simulink model "Have_Loop_Current"  (Simulink 7.5)
settings: Solver=ode45  StartTime=0.0  StopTime=10  RelTol=1e-3
libraries: powerlib x28, simulink x2, powerlib_extras x2
settings Model: Creator=lm  LastModifiedBy=lm

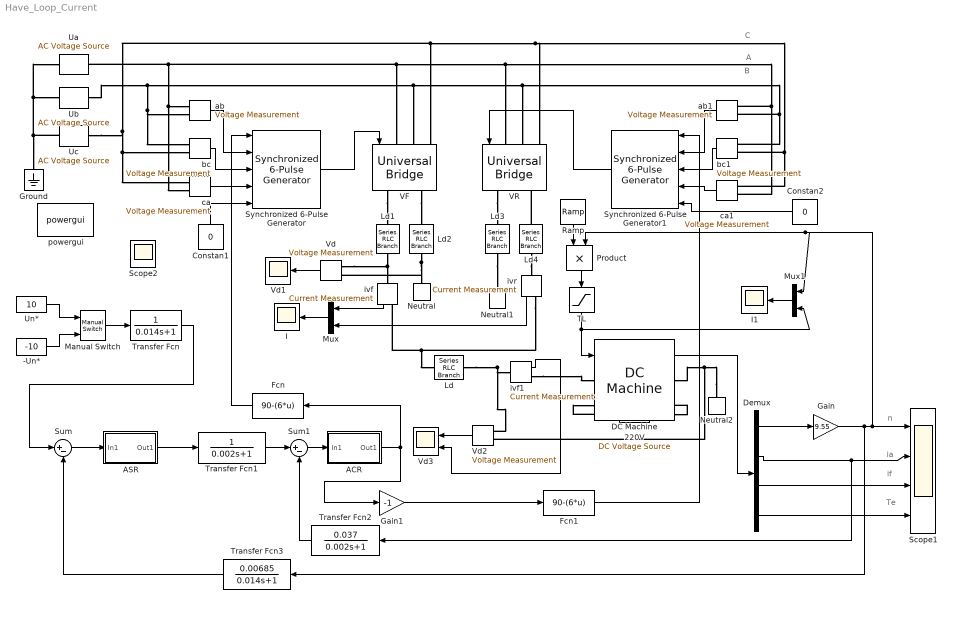
== system Have_Loop_Current ==
  note: A
  note: B
  note: C
  note: n
  note: ia
  note: if
  note: Te
  -Un* : Constant  Value=-10  OutDataType=fixdt(1, 16)  OutScaling=2^0
  220V : powerlib/Electrical Sources/DC Voltage Source  DialogController=POWERSYS.PowerSysDialog  SystemSampleTime=-1  Amplitude=220  Measurements=None
  ACR : Subsystem
  ASR : Subsystem
  Constan1 : Constant  Value=0  OutDataType=fixdt(1, 16)  OutScaling=2^0
  Constan2 : Constant  Value=0  OutDataType=fixdt(1, 16)  OutScaling=2^0
  DC Machine : powerlib/Machines/DC Machine  DialogController=POWERSYS.PowerSysDialog  SystemSampleTime=-1  PresetModel=No  MechanicalLoad=Torque TL  FieldType=Wound  ShowDetailedParameters=on  RLa="[ 0.21  0.000543]"  RLf="[ 14.7  0]"  Laf=0.084  MachineConstant=Torque constant (N.m/A)  Ke=1.8  Kt=1.8  J=2.29  Bm=0  Tf=0  w0=1  Ifinit=1  TsPowergui=0  TsBlock=-1
      settings: AttributesFormatString=\n
  Demux : Demux
  Fcn : Fcn  Expr=90-(6*u)
  Fcn1 : Fcn  Expr=90-(6*u)
  Gain : Gain  Gain=9.55  ParameterDataType=fixdt(1, 16)  ParameterScaling=2^0  OutDataType=fixdt(1, 16)  OutScaling=2^0
  Gain1 : Gain  Gain=-1  ParameterDataType=fixdt(1, 16)  ParameterScaling=2^0  OutDataType=fixdt(1, 16)  OutScaling=2^0
  Ground : powerlib/Elements/Ground  DialogController=POWERSYS.PowerSysDialog  PhysicalDomain=powersysdomain  SubClassName=unknown  LeftPortType=p1  RightPortType=p1  LConnTagsString=a
  I : Scope
  I1 : Scope
      settings: SaveName=ScopeData5
  Ld : powerlib/Elements/Series RLC Branch  DialogController=POWERSYS.PowerSysDialog  PhysicalDomain=powersysdomain  SubClassName=unknown  LeftPortType=p1  RightPortType=p1  LConnTagsString=__new0  RConnTagsString=__new0  BranchType=RL  Resistance=0.002  Inductance=0.015  SetiL0=off  InitialCurrent=0  Capacitance=1e-6  Setx0=off  InitialVoltage=0  Measurements=None
  Ld{1..4} (4 alike) : powerlib/Elements/Series RLC Branch  DialogController=POWERSYS.PowerSysDialog  PhysicalDomain=powersysdomain  SubClassName=unknown  LeftPortType=p1  RightPortType=p1  LConnTagsString=__new0  RConnTagsString=__new0  BranchType=L  Resistance=1  Inductance=2e-3  SetiL0=off  InitialCurrent=0  Capacitance=1e-6  Setx0=off  InitialVoltage=0  Measurements=None
  Manual Switch : simulink/Signal Routing/Manual Switch  SystemSampleTime=-1  sw=0  action=0  varsize=off
  Mux : Mux  Inputs=2
  Mux1 : Mux  Inputs=2
  Neutral : powerlib/Elements/Neutral  DialogController=POWERSYS.PowerSysDialog  PhysicalDomain=powersysdomain  SubClassName=unknown  LeftPortType=p1  RightPortType=p1  LConnTagsString=a  NodeNumber=10
  Neutral1 : powerlib/Elements/Neutral  DialogController=POWERSYS.PowerSysDialog  PhysicalDomain=powersysdomain  SubClassName=unknown  LeftPortType=p1  RightPortType=p1  LConnTagsString=a  NodeNumber=10
  Neutral2 : powerlib/Elements/Neutral  DialogController=POWERSYS.PowerSysDialog  PhysicalDomain=powersysdomain  SubClassName=unknown  LeftPortType=p1  RightPortType=p1  LConnTagsString=a  NodeNumber=10
  Product : Product  OutDataType=fixdt(1, 16)  OutScaling=2^0  RndMeth=Zero
  Ramp : simulink/Sources/Ramp  SystemSampleTime=-1  slope=10000  start=2.2  X0=0
  Scope1 : Scope  NumInputPorts=4
      settings: YMin=1275~-20~14.966~-25  YMax=1475~140~14.966~175
  Scope2 : Scope
      settings: YMin=-10  YMax=10  SaveName=ScopeData2
  Sum : Sum  Inputs=|+-  OutDataType=fixdt(1, 16)  OutScaling=2^0
  Sum1 : Sum  Inputs=|+-  OutDataType=fixdt(1, 16)  OutScaling=2^0
  Synchronized 6-Pulse Generator : powerlib_extras/Control  Blocks/Synchronized 6-Pulse Generator  DialogController=POWERSYS.PowerSysDialog  SystemSampleTime=-1  freq=60  pwidth=10  Double_Pulse=off
  Synchronized 6-Pulse Generator1 : powerlib_extras/Control  Blocks/Synchronized 6-Pulse Generator  DialogController=POWERSYS.PowerSysDialog  SystemSampleTime=-1  freq=60  pwidth=10  Double_Pulse=off
  TL : Saturate  UpperLimit=160  LowerLimit=-160  OutDataType=fixdt(1, 16)  OutScaling=2^0
  Transfer Fcn : TransferFcn  Denominator=[0.014 1]
  Transfer Fcn1 : TransferFcn  Denominator=[0.002 1]
  Transfer Fcn2 : TransferFcn  Numerator=[0.037]  Denominator=[0.002 1]
  Transfer Fcn3 : TransferFcn  Numerator=[0.00685]  Denominator=[0.014 1]
  Ua : powerlib/Electrical Sources/AC Voltage Source  DialogController=POWERSYS.PowerSysDialog  SystemSampleTime=-1  Amplitude=160  Phase=0  Frequency=50  SampleTime=0  Measurements=None
  Ub : powerlib/Electrical Sources/AC Voltage Source  DialogController=POWERSYS.PowerSysDialog  SystemSampleTime=-1  Amplitude=160  Phase=-120  Frequency=50  SampleTime=0  Measurements=None
  Uc : powerlib/Electrical Sources/AC Voltage Source  DialogController=POWERSYS.PowerSysDialog  SystemSampleTime=-1  Amplitude=160  Phase=-240  Frequency=50  SampleTime=0  Measurements=None
  Un* : Constant  Value=10  OutDataType=fixdt(1, 16)  OutScaling=2^0
  VF : powerlib/Power Electronics/Universal Bridge  DialogController=POWERSYS.PowerSysDialog  SystemSampleTime=-1  Arms=3  SnubberResistance=1e5  SnubberCapacitance=inf  Device=Thyristors  Ron=1e-3  Lon=0  ForwardVoltages="[  0  0  ]"  ForwardVoltage=0  GTOparameters=[ 10e-6 , 20e-6 ]  IGBTparameters=[ 1e-6 , 2e-6 ]  Measurements=None  Measurements_2=None  converterType=Rectifier
  VR : powerlib/Power Electronics/Universal Bridge  DialogController=POWERSYS.PowerSysDialog  SystemSampleTime=-1  Arms=3  SnubberResistance=1e5  SnubberCapacitance=inf  Device=Thyristors  Ron=1e-3  Lon=0  ForwardVoltages="[  0  0  ]"  ForwardVoltage=0  GTOparameters=[ 10e-6 , 20e-6 ]  IGBTparameters=[ 1e-6 , 2e-6 ]  Measurements=None  Measurements_2=None  converterType=Rectifier
  Vd : powerlib/Measurements/Voltage Measurement  DialogController=POWERSYS.PowerSysDialog  SystemSampleTime=-1  PhasorSimulation=off  OutputType=Complex  PSBequivalent=0
  Vd1 : Scope
      settings: YMin=-400  YMax=500  SaveName=ScopeData3
  Vd2 : powerlib/Measurements/Voltage Measurement  DialogController=POWERSYS.PowerSysDialog  SystemSampleTime=-1  PhasorSimulation=off  OutputType=Complex  PSBequivalent=0
  Vd3 : Scope  NumInputPorts=2
      settings: YMin=-5~-5  YMax=5~5  SaveName=ScopeData4
  ab : powerlib/Measurements/Voltage Measurement  DialogController=POWERSYS.PowerSysDialog  SystemSampleTime=-1  PhasorSimulation=off  OutputType=Complex  PSBequivalent=0
  ab1 : powerlib/Measurements/Voltage Measurement  DialogController=POWERSYS.PowerSysDialog  SystemSampleTime=-1  PhasorSimulation=off  OutputType=Complex  PSBequivalent=0
  bc : powerlib/Measurements/Voltage Measurement  DialogController=POWERSYS.PowerSysDialog  SystemSampleTime=-1  PhasorSimulation=off  OutputType=Complex  PSBequivalent=0
  bc1 : powerlib/Measurements/Voltage Measurement  DialogController=POWERSYS.PowerSysDialog  SystemSampleTime=-1  PhasorSimulation=off  OutputType=Complex  PSBequivalent=0
  ca : powerlib/Measurements/Voltage Measurement  DialogController=POWERSYS.PowerSysDialog  SystemSampleTime=-1  PhasorSimulation=off  OutputType=Complex  PSBequivalent=0
  ca1 : powerlib/Measurements/Voltage Measurement  DialogController=POWERSYS.PowerSysDialog  SystemSampleTime=-1  PhasorSimulation=off  OutputType=Complex  PSBequivalent=0
  ivf : powerlib/Measurements/Current Measurement  DialogController=POWERSYS.PowerSysDialog  SystemSampleTime=-1  PhasorSimulation=off  OutputType=Complex  PSBequivalent=0
  ivf1 : powerlib/Measurements/Current Measurement  DialogController=POWERSYS.PowerSysDialog  SystemSampleTime=-1  PhasorSimulation=off  OutputType=Complex  PSBequivalent=0
  ivr : powerlib/Measurements/Current Measurement  DialogController=POWERSYS.PowerSysDialog  SystemSampleTime=-1  PhasorSimulation=off  OutputType=Complex  PSBequivalent=0
  powergui : powerlib/powergui  Priority=1  SystemSampleTime=-1  SimulationMode=Discrete  SampleTime=50e-6  frequency=60  SPID=off  DisableSnubberDevices=off  DisableRonSwitches=off  DisableVfSwitches=off  SwTol=0  Interpol=off  frequencyindice=0  echomessages=off  HookPort=off  DisplayEquations=off  FunctionMessages=off  EnableUseOfTLC=off  x0status=blocks  RestoreLinks=warning  ResistiveCurrentMeasurement=off  Ylog=off  Xlog=on  ShowGrid=off  save=off  variable=ZData  ZoomFFT=off  StartTime=0.0  cycles=1  DisplayStyle=1  FreqAxis=off  MaxFrequency=1000  frequencyindicesteady=1  display=off  methode=off
  wires:
  ab/1 -> Synchronized 6-Pulse Generator/2
  bc/1 -> Synchronized 6-Pulse Generator/3
  ca/1 -> Synchronized 6-Pulse Generator/4
  Constan1/1 -> Synchronized 6-Pulse Generator/5
  Synchronized 6-Pulse Generator/1 -> VF/1
  Synchronized 6-Pulse Generator1/1 -> VR/1
  ab1/1 -> Synchronized 6-Pulse Generator1/2
  bc1/1 -> Synchronized 6-Pulse Generator1/3
  ca1/1 -> Synchronized 6-Pulse Generator1/4
  Constan2/1 -> Synchronized 6-Pulse Generator1/5
  Un*/1 -> Manual Switch/1
  -Un*/1 -> Manual Switch/2
  Manual Switch/1 -> Transfer Fcn/1
  DC Machine/1 -> Demux/1
  Demux/1 -> Gain/1
  Gain/1 -> Transfer Fcn3/1, Scope1/1, Product/2, Mux1/1
  Demux/2 -> Scope1/2, Transfer Fcn2/1
  Demux/3 -> Scope1/3
  Demux/4 -> Scope1/4
  Transfer Fcn/1 -> Sum/1
  ASR/1(Out1) -> Transfer Fcn1/1
  Sum/1 -> ASR/1(In1)
  Transfer Fcn1/1 -> Sum1/1
  Sum1/1 -> ACR/1(In1)
  ACR/1(Out1) -> Fcn/1, Gain1/1
  Fcn/1 -> Synchronized 6-Pulse Generator/1
  Gain1/1 -> Fcn1/1
  Fcn1/1 -> Synchronized 6-Pulse Generator1/1
  Transfer Fcn2/1 -> Sum1/2
  Transfer Fcn3/1 -> Sum/2
  ivf/1 -> Mux/1
  ivr/1 -> Mux/2
  Mux/1 -> I/1
  Vd/1 -> Vd1/1
  Vd2/1 -> Vd3/1
  ivf1/1 -> Vd3/2
  TL/1 -> DC Machine/1, Mux1/2
  Ramp/1 -> Product/1
  Product/1 -> TL/1
  Mux1/1 -> I1/1
  connections:
  Uc/LConn1 -- Ground/LConn1 -- Ub/LConn1 -- Ua/LConn1
  220V/RConn1 -- DC Machine/LConn2
  220V/LConn1 -- DC Machine/RConn2
  VF/LConn1 -- ab1/LConn1 -- ca1/LConn2 -- VR/LConn1 -- Ua/RConn1 -- ab/LConn1 -- ca/LConn2
  Ub/RConn1 -- ab/LConn2 -- bc/LConn1 -- VF/LConn2 -- ab1/LConn2 -- bc1/LConn1 -- VR/LConn2
  VF/LConn3 -- bc1/LConn2 -- ca1/LConn1 -- VR/LConn3 -- Uc/RConn1 -- bc/LConn2 -- ca/LConn1
  VF/RConn1 -- Ld1/LConn1
  VF/RConn2 -- Ld2/LConn1
  VR/RConn1 -- Ld3/LConn1
  Ld4/LConn1 -- VR/RConn2
  Vd/LConn1 -- ivf/LConn1 -- Ld1/RConn1
  ivr/RConn1 -- ivf/RConn1 -- Ld/LConn1
  Ld/RConn1 -- Vd2/LConn1 -- ivf1/LConn1
  Neutral/LConn1 -- Ld2/RConn1 -- Vd/LConn2
  Neutral2/LConn1 -- DC Machine/RConn1 -- Vd2/LConn2
  Ld4/RConn1 -- ivr/LConn1
  ivf1/RConn1 -- DC Machine/LConn1
  Ld3/RConn1 -- Neutral1/LConn1

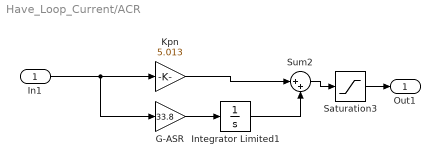
== system Have_Loop_Current/ACR ==
  In1 : Inport
  G-ASR : Gain  Gain=33.8  ParameterDataType=fixdt(1, 16)  ParameterScaling=2^0  OutDataType=fixdt(1, 16)  OutScaling=2^0
  Integrator Limited1 : Integrator  LimitOutput=on  UpperSaturationLimit=12  LowerSaturationLimit=-12
  Kpn : Gain  Gain=5.013  ParameterDataType=fixdt(1, 16)  ParameterScaling=2^0  OutDataType=fixdt(1, 16)  OutScaling=2^0
  Saturation3 : Saturate  UpperLimit=10  LowerLimit=-10  OutDataType=fixdt(1, 16)  OutScaling=2^0
  Sum2 : Sum  Inputs=|++  OutDataType=fixdt(1, 16)  OutScaling=2^0
  Out1 : Outport
  wires:
  Saturation3/1 -> Out1/1
  In1/1 -> G-ASR/1, Kpn/1
  Integrator Limited1/1 -> Sum2/2
  Kpn/1 -> Sum2/1
  G-ASR/1 -> Integrator Limited1/1
  Sum2/1 -> Saturation3/1

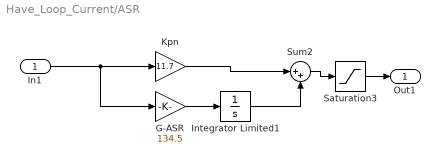
== system Have_Loop_Current/ASR ==
  In1 : Inport
  G-ASR : Gain  Gain=134.5  ParameterDataType=fixdt(1, 16)  ParameterScaling=2^0  OutDataType=fixdt(1, 16)  OutScaling=2^0
  Integrator Limited1 : Integrator  LimitOutput=on  UpperSaturationLimit=12  LowerSaturationLimit=-12
  Kpn : Gain  Gain=11.7  ParameterDataType=fixdt(1, 16)  ParameterScaling=2^0  OutDataType=fixdt(1, 16)  OutScaling=2^0
  Saturation3 : Saturate  UpperLimit=10  LowerLimit=-10  OutDataType=fixdt(1, 16)  OutScaling=2^0
  Sum2 : Sum  Inputs=|++  OutDataType=fixdt(1, 16)  OutScaling=2^0
  Out1 : Outport
  wires:
  Sum2/1 -> Saturation3/1
  G-ASR/1 -> Integrator Limited1/1
  Kpn/1 -> Sum2/1
  Integrator Limited1/1 -> Sum2/2
  In1/1 -> Kpn/1, G-ASR/1
  Saturation3/1 -> Out1/1
